simulink model "VCU_2023"  (Simulink 10.1)
settings: Solver=FixedStepDiscrete  StartTime=0.0  StopTime=10.0  FixedStep=0.001  RelTol=1e-3  EnableMultiTasking=on
PreLoadFcn:
  | try
  | MDL_setup;
  | catch
  | end
InitFcn:
  | EcoCoder_PreCheckLic();
undefined symbols (not defined in the file): APPS_max, APPS_min, BRK_TH, DiscIntNeverNeededParam
libraries: CoderSF_BSW_Libs x156, simulink x11
(part 1 of 2)
settings Model: Creator=HXL  LastModifiedBy=ecuri
settings Model: SuppressorTable=|
  | <?xml version="1.0" encoding="UTF-8" standalone="yes" ?>
  | <!DOCTYPE boost_serialization>
  | <boost_serialization signature="serialization::archive" version="17">
  | <DiagnosticSuppressor class_id="0" tracking_level="0" version="6">
  | 	<Table class_id="1" tracking_level="0" version="0">
  | 		<count>4</count>
  | 		<bucket_count>8</bucket_count>
  | 		<item_version>0</item_version>
  | 		<item class_id="2" tracking_level="0" version="0">
  | 			<first class_id="3" tracking_level="0" version="6">
  | 				<Source class_id="4" tracking_level="0" version="0">
  | 					<count>1</count>
  | 					<item_version>0</item_version>
  | 					<item>VCU_2023/Subsystem/CAN/Triggered Subsystem/N_R_Dec | M_R_Dec/Extract Bits1</item>
  | 				</Source>
  | 			</first>
  | 			<second class_id="5" tracking_level="0" version="6">
  | 				<SuppressedData class_id="6" tracking_level="0" version="0">
  | 					<count>2</count>
  | 					<bucket_count>8</bucket_count>
  | 					<item_version>0</item_version>
  | 					<item class_id="7" tracking_level="0" version="0">
  | 						<first class_id="8" tracking_level="0" version="6">
  | 							<ID>Simulink:DataType:WarningOverFlowDetected</ID>
  | 							<Cause>
  | 								<Source>
  | 									<count>0</count>
  | 									<item_version>0</item_version>
  | 								</Source>
  | 							</Cause>
  | 						</first>
  | 						<second class_id="9" tracking_level="0" version="6">
  | 							<Comment></Comment>
  | 							<User></User>
  | 							<LastModified class_id="10" tracking_level="0" version="0">
  | 								<ptime_date class_id="11" tracking_level="0" version="0">
  | 									<date>20160608</date>
  | 								</ptime_date>
  | 								<ptime_time_duration class_id="12" tracking_level="0" version="1">
  | 									<is_special>0</is_special>
  | 									<time_duration_hours>15</time_duration_hours>
  | 									<time_duration_minutes>43</time_duration_minutes>
  | 									<time_duration_seconds>6</time_duration_seconds>
  | 									<time_duration_fractional_seconds>0</time_duration_fractional_seconds>
  | 								</ptime_time_duration>
  | 							</LastModified>
  | 							<SuppressionType>1</SuppressionType>
  | 						</second>
  | 					</item>
  | 					<item>
  | 						<first>
  | 							<ID>SimulinkFixedPoint:util:Overflowoccurred</ID>
  | 							<Cause>
  | 								<Source>
  | 									<count>0</count>
  | 									<item_version>0</item_version>
  | 								</Source>
  | 							</Cause>
  | 						</first>
  | 						<second>
  | 							<Comment></Comment>
  | 							<User></User>
  | 							<LastModified>
  | 								<ptime_date>
  | 									<date>20160608</date>
  | 								</ptime_date>
  | 								<ptime_time_duration>
  | 									<is_special>0</is_special>
  | 									<time_duration_hours>15</time_duration_hours>
  | 									<time_duration_minutes>43</time_duration_minutes>
  | 									<time_duration_seconds>6</time_duration_seconds>
  | 									<time_duration_fractional_seconds>0</time_duration_fractional_seconds>
  | 								</ptime_time_duration>
  | 							</LastModified>
  | 							<SuppressionType>1</SuppressionType>
  | 						</second>
  | 					</item>
  | 				</SuppressedData>
  | 			</second>
  | 		</item>
  | 		<item>
  | 			<first>
  | 				<Source>
  | 					<count>1</count>
  | 					<item_version>0</item_version>
  | 					<item>VCU_2023/Subsystem/CAN/Triggered Subsystem/N_R_Dec | M_R_Dec/Extract Bits</item>
  | 				</Source>
  | 			</first>
  | 			<second>
  | 				<SuppressedData>
  | 					<count>2</count>
  | 					<bucket_count>8</bucket_count>
  | 					<item_version>0</item_version>
  | 					<item>
  | 						<first>
  | 							<ID>Simulink:DataType:WarningOverFlowDetected</ID>
  | 							<Cause>
  | 								<Source>
  | 									<count>0</count>
  | 									<item_version>0</item_version>
  | 								</Source>
  | 							</Cause>
  | 						</first>
  | 						<second>
  | 							<Comment></Comment>
  | 							<User></User>
  | 							<LastModified>
  | 								<ptime_date>
  | 									<date>20160608</date>
  | 								</ptime_date>
  | 								<ptime_time_duration>
  | 									<is_special>0</is_special>
  | 									<time_duration_hours>15</time_duration_hours>
  | 									<time_duration_minutes>43</time_duration_minutes>
  | 									<time_duration_seconds>6</time_duration_seconds>
  | 									<time_duration_fractional_seconds>0</time_duration_fractional_seconds>
  | 								</ptime_time_duration>
  | 							</LastModified>
  | 							<SuppressionType>1</SuppressionType>
  | 						</second>
  | 					</item>
  | 					<item>
  | 						<first>
  | 							<ID>SimulinkFixedPoint:util:Overflowoccurred</ID>
  | 							<Cause>
  | 								<Source>
  | 									<count>0</count>
  | 									<item_version>0</item_version>
  | 								</Source>
  | 							</Cause>
  | 						</first>
  | 						<second>
  | 							<Comment></Comment>
  | 							<User></User>
  | 							<LastModified>
  | 								<ptime_date>
  | 									<date>20160608</date>
  | 								</ptime_date>
  | 								<ptime_time_duration>
  | 									<is_special>0</is_special>
  | 									<time_duration_hours>15</time_duration_hours>
  | 									<time_duration_minutes>43</time_duration_minutes>
  | 									<time_duration_seconds>6</time_duration_seconds>
  | 									<time_duration_fractional_seconds>0</time_duration_fractional_seconds>
  | 								</ptime_time_duration>
  | 							</LastModified>
  | 							<SuppressionType>1</SuppressionType>
  | 						</second>
  | 					</item>
  | 				</SuppressedData>
  | 			</second>
  | 		</item>
  | 		<item>
  | 			<first>
  | 				<Source>
  | 					<count>1</count>
  | 					<item_version>0</item_version>
  | 					<item>VCU_2023/Subsystem/CAN/Triggered Subsystem/N_R_Acc | M R_Acc/Extract Bits1</item>
  | 				</Source>
  | 			</first>
  | 			<second>
  | 				<SuppressedData>
  | 					<count>2</count>
  | 					<bucket_count>8</bucket_count>
  | 					<item_version>0</item_version>
  | 					<item>
  | 						<first>
  | 							<ID>Simulink:DataType:WarningOverFlowDetected</ID>
  | 							<Cause>
  | 								<Source>
  | 									<count>0</count>
  | 									<item_version>0</item_version>
  | 								</Source>
  | 							</Cause>
  | 						</first>
  | 						<second>
  | 							<Comment></Comment>
  | 							<User></User>
  | 							<LastModified>
  | 								<ptime_date>
  | 									<date>20160608</date>
  | 								</ptime_date>
  | 								<ptime_time_duration>
  | 									<is_special>0</is_special>
  | 									<time_duration_hours>15</time_duration_hours>
  | 									<time_duration_minutes>43</time_duration_minutes>
  | 									<time_duration_seconds>6</time_duration_seconds>
  | 									<time_duration_fractional_seconds>0</time_duration_fractional_seconds>
  | 								</ptime_time_duration>
  | 							</LastModified>
  | 							<SuppressionType>1</SuppressionType>
  | 						</second>
  | 					</item>
  | 					<item>
  | 						<first>
  | 							<ID>SimulinkFixedPoint:util:Overflowoccurred</ID>
  | 							<Cause>
  | 								<Source>
  | 									<count>0</count>
  | 									<item_version>0</item_version>
  | 								</Source>
  | 							</Cause>
  | 						</first>
  | 						<second>
  | 							<Comment></Comment>
  | 							<User></User>
  | 							<LastModified>
  | 								<ptime_date>
  | 									<date>20160608</date>
  | 								</ptime_date>
  | 								<ptime_time_duration>
  | 									<is_special>0</is_special>
  | 									<time_duration_hours>15</time_duration_hours>
  | 									<time_duration_minutes>43</time_duration_minutes>
  | 									<time_duration_seconds>6</time_duration_seconds>
  | 									<time_duration_fractional_seconds>0</time_duration_fractional_seconds>
  | 								</ptime_time_duration>
  | 							</LastModified>
  | 							<SuppressionType>1</SuppressionType>
  | 						</second>
  | 					</item>
  | 				</SuppressedData>
  | 			</second>
  | 		</item>
  | 		<item>
  | 			<first>
  | 				<Source>
  | 					<count>1</count>
  | 					<item_version>0</item_version>
  | 					<item>VCU_2023/Subsystem/CAN/Triggered Subsystem/N_R_Acc | M R_Acc/Extract Bits</item>
  | 				</Source>
  | 			</first>
  | 			<second>
  | 				<SuppressedData>
  | 					<count>2</count>
  | 					<bucket_count>8</bucket_count>
  | 					<item_version>0</item_version>
  | 					<item>
  | 						<first>
  | 							<ID>Simulink:DataType:WarningOverFlowDetected</ID>
  | 							<Cause>
  | 								<Source>
  | 									<count>0</count>
  | 									<item_version>0</item_version>
  | 								</Source>
  | 							</Cause>
  | 						</first>
  | 						<second>
  | 							<Comment></Comment>
  | 							<User></User>
  | 							<LastModified>
  | 								<ptime_date>
  | 									<date>20160608</date>
  | 								</ptime_date>
  | 								<ptime_time_duration>
  | 									<is_special>0</is_special>
  | 									<time_duration_hours>15</time_duration_hours>
  | 									<time_duration_minutes>43</time_duration_minutes>
  | 									<time_duration_seconds>6</time_duration_seconds>
  | 									<time_duration_fractional_seconds>0</time_duration_fractional_seconds>
  | 								</ptime_time_duration>
  | 							</LastModified>
  | 							<SuppressionType>1</SuppressionType>
  | 						</second>
  | 					</item>
  | 					<item>
  | 						<first>
  | 							<ID>SimulinkFixedPoint:util:Overflowoccurred</ID>
  | 							<Cause>
  | 								<Source>
  | 									<count>0</count>
  | 									<item_version>0</item_version>
  | 								</Source>
  | 							</Cause>
  | 						</first>
  | 						<second>
  | 							<Comment></Comment>
  | 							<User></User>
  | 							<LastModified>
  | 								<ptime_date>
  | 									<date>20160608</date>
  | 								</ptime_date>
  | 								<ptime_time_duration>
  | 									<is_special>0</is_special>
  | 									<time_duration_hours>15</time_duration_hours>
  | 									<time_duration_minutes>43</time_duration_minutes>
  | 									<time_duration_seconds>6</time_duration_seconds>
  | 									<time_duration_fractional_seconds>0</time_duration_fractional_seconds>
  | 								</ptime_time_duration>
  | 							</LastModified>
  | 							<SuppressionType>1</SuppressionType>
  | 						</second>
  | 					</item>
  | 				</SuppressedData>
  | 			</second>
  | 		</item>
  | 	</Table>
  | </DiagnosticSuppressor>
  | 
  | </boost_serialization>
  | 
  | </boost_serialization>
settings DataIOCC: ExternalInput=InputData  SaveFormat=Structure  SignalLoggingSaveFormat=ModelDataLogs  SaveOutput=off  SignalLogging=off  DSMLogging=off  SaveTime=off
settings OptimizationCC: DefaultParameterBehavior=Inlined  InlineInvariantSignals=on  EnhancedBackFolding=on  StrengthReduction=on  EnableMemcpy=off  PassReuseOutputArgsAs=Individual arguments  ExpressionDepthLimit=2147483647  EfficientFloat2IntCast=on  LifeSpan=1  SimCompilerOptimization=on  OptimizeBlockOrder=speed  DifferentSizesBufferReuse=on  EfficientTunableParamExpr=on
settings DebuggingCC: AlgebraicLoopMsg=none  ArtificialAlgebraicLoopMsg=none  SaveWithDisabledLinksMsg=none  SaveWithParameterizedLinksMsg=none  CheckSSInitialOutputMsg=off  SignalResolutionControl=TryResolveAll  BlockPriorityViolationMsg=error  MinStepSizeMsg=none  InheritedTsInSrcMsg=none  MultiTaskDSMMsg=none  MultiTaskCondExecSysMsg=none  MultiTaskRateTransMsg=warning  TasksWithSamePriorityMsg=none  SigSpecEnsureSampleTimeMsg=none  IntegerOverflowMsg=error  Int32ToFloatConvMsg=none  ParameterPrecisionLossMsg=none  ParameterTunabilityLossMsg=none  FixptConstOverflowMsg=error  FcnCallInpInsideContextMsg=warning  UnconnectedInputMsg=error  UnconnectedOutputMsg=error  UnconnectedLineMsg=error  FrameProcessingCompatibilityMsg=none  BusObjectLabelMismatch=none  RootOutportRequireBusObject=none  UnknownTsInhSupMsg=none  ModelReferenceDataLoggingMessage=none  OperatingPointInterfaceChecksumMismatchMsg=none  SFUnusedDataAndEventsDiag=none  SFUnexpectedBacktrackingDiag=none  SFInvalidInputDataAccessInChartInitDiag=none  SFNoUnconditionalDefaultTransitionDiag=none  SFTransitionOutsideNaturalParentDiag=none  SFUnreachableExecutionPathDiag=none  IntegerSaturationMsg=error
settings HardwareCC: ProdLargestAtomicInteger=Long  ProdLargestAtomicFloat=Double  ProdIntDivRoundTo=Zero  ProdEndianess=BigEndian  ProdHWDeviceType=Freescale->MPC55xx  TargetIntDivRoundTo=Zero  TargetEndianess=BigEndian  TargetHWDeviceType=Freescale->MPC55xx
settings ModelReferenceCC: UpdateModelReferenceTargets=Force  ModelReferenceNumInstancesAllowed=Single
settings SFSimCC: SFSimEcho=off  SimBuildMode=sf_make_clean  MATLABDynamicMemAlloc=off
settings RTWCC: Description=Ecotrons MPC5xxx  SystemTargetFile=MPC5644A.tlc  GenerateMakefile=off  TemplateMakefile=ert_default_tmf  RTWVerbose=off  RetainRTWFile=on  RTWCompilerOptimization=on
settings CodeAppCC: IgnoreCustomStorageClasses=off  OperatorAnnotations=on  CustomSymbolStrGlobalVar=$N$M  CustomSymbolStrType=$N$M  CustomSymbolStrFcn=$N$M  CustomSymbolStrFcnArg=$N$M  CustomSymbolStrBlkIO=$N$M  CustomSymbolStrMacro=$N$M  StateflowObjectComments=off  InternalIdentifier=Classic
settings STFCustomTargetCC: CodeReplacementLibrary=ANSI_C  UtilityFuncGeneration=Shared location  MultiwordLength=256  IncludeMdlTerminateFcn=off  CombineOutputUpdateFcns=on  SuppressErrorStatus=on  ERTCustomFileBanners=on  SupportNonFinite=off  SupportComplex=off  SupportContinuousTime=off  SupportNonInlinedSFcns=off  MATLABClassNameForMDSCustomization=Simulink.SoftwareTarget.ERTCustomization  GRTInterface=off  SystemTargetFile=MPC5644A.tlc
settings ERTTargetCC: CodeReplacementLibrary=ANSI_C  UtilityFuncGeneration=Shared location  ParMdlRefBuildCompliant=off  CompOptLevelCompliant=off  ConcurrentExecutionCompliant=off  IncludeMdlTerminateFcn=off  SuppressErrorStatus=on  SupportNonFinite=off  SupportComplex=off  RemoveResetFunc=off  ModelStepFunctionPrototypeControlCompliant=off  CPPClassGenCompliant=off  UseToolchainInfoCompliant=off  GenerateASAP2=on  InlinedParameterPlacement=NonHierarchical  ERTCustomFileTemplate=MPC5644A_file_process.tlc  ERTFilePackagingFormat=Compact  PreserveIfCondition=on  ConvertIfToSwitch=off  PreserveExternInFcnDecls=off  SuppressUnreachableDefaultCases=off
settings CustomProperty: DataType=string  Value=EV2274A
settings EnumStrPairs: String=Removed
settings ConfigComp: DVMaxProcessTime=3600  DVDisplayUnsatisfiableObjectives=on  DVModelCoverageObjectives=MCDC  DVMaxTestCaseSteps=500  DVTestSuiteOptimization=CombinedObjectives  DVDetectActiveLogic=on

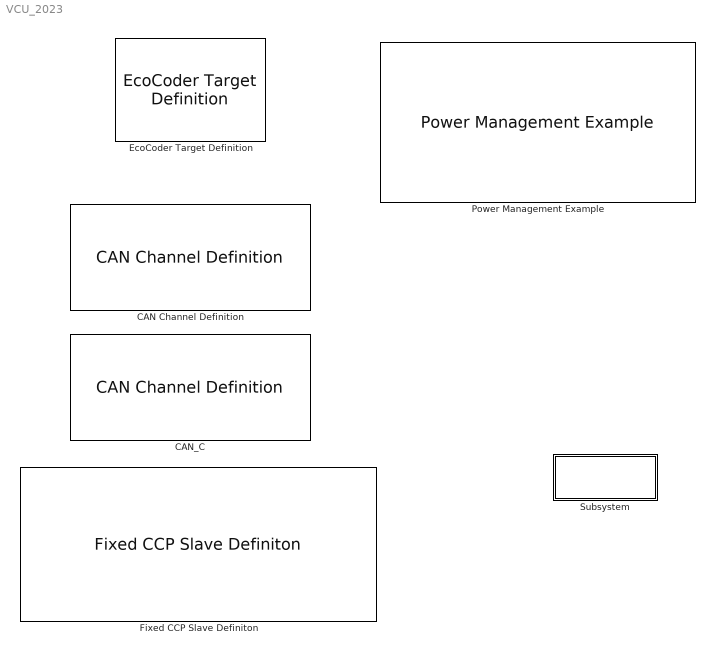
== system VCU_2023 ==
  CAN Channel Definition : CoderSF_BSW_Libs/CAN/CAN Channel Definition  channel=CAN_A  can_en=on  can_idfilter=off  can_rxextended=off  can_rxMask=hex2dec('7ff')  can_rxID=hex2dec('100')  can_baudrateIndex=500  can_txbuffer_size=30  can_rxbuffer_size=1  can_en_fd=off  nominalSamplePoint=7500  can_baudrateIndex_data=500  fastSamplePoint=7500  canfd_txbuffer_size=5  EcoCoderBlockID=C001_CANDef
  CAN_C : CoderSF_BSW_Libs/CAN/CAN Channel Definition  channel=CAN_C  can_en=on  can_idfilter=off  can_rxextended=off  can_rxMask=hex2dec('7ff')  can_rxID=hex2dec('100')  can_baudrateIndex=500  can_txbuffer_size=30  can_rxbuffer_size=1  can_en_fd=off  nominalSamplePoint=7500  can_baudrateIndex_data=500  fastSamplePoint=7500  canfd_txbuffer_size=5  EcoCoderBlockID=C001_CANDef
  EcoCoder Target Definition : CoderSF_BSW_Libs/EcoCoder Target Definition  targetECU=EV2274A  EcoCoderBlockID=T001_Target  enNoTriggerCall=on  flgBlockReduction=on  flgShowDebugDisp=off  flgDisTargetOutFIleCounter=off  flgClearAllOldFiles=on  tc275_cal_len=hex2dec('00008000')  internal_flash=[hex2dec('00020000'),hex2dec('000E0000')]  cal_rom_phy=[hex2dec('00010000'),hex2dec('00002000')]  cal_ram_wp=[hex2dec('4000F000'),hex2dec('00002000')]  cal_ram_msm=[hex2dec('40000000'),hex2dec('00002000')]  var_ram_wp=[hex2dec('40002000'),hex2dec('0000D000')]  write_back_fixed_ram=[hex2dec('40011000'),hex2dec('00001000')]  write_back_unfixed_ram=[hex2dec('40012000'),hex2dec('00001000')]  stack=[hex2dec('40013000'),hex2dec('00001000')]
      settings: AttributesFormatString=Target :%<targetECU>
  Fixed CCP Slave Definiton : CoderSF_BSW_Libs/CCP/Fixed CCP Slave Definiton  ccpType=Configurable  ccp_enSet=on  ccp_disASW=on  channel=CAN_A  stationaddressSet=hex2dec('0112')  croidSet=hex2dec('100')  dtoidSet=hex2dec('101')  daqidSet=[hex2dec('101') hex2dec('101') hex2dec('101') hex2dec('102')]  daqpidSet=[hex2dec('0') hex2dec('3C') hex2dec('78') hex2dec('0')]  daqlenSet=[hex2dec('0') hex2dec('20') hex2dec('30') hex2dec('30')]  daqperSet=[5 20 100 0]  EcoCoderBlockID=C002_CCPConf
  Power Management Example : CoderSF_BSW_Libs/System Management Blocks/Power Management Example  Priority=1  flgKeyFromIn=off  tKeyOffDelaySet=0.5  flgResetSWEnSet=1  tDbncKeyOffFallSet=0.1  tDbncKeyOffRiseSet=0.1  facAd2VoltSet=109/27846  uKeyOffThrSet=1  uKeyOnHystSet=1  flgCANRxLiveCheckEn=0  flgEnPwrDwnFailReset=0  flgNVMEn=on  tShtDwnWait=500  flgPwrDwnByEdgeTrigger=off  EcoCoderBlockID=PME001_Def
      settings: AttributesFormatString=Priority:%<Priority>
  Subsystem : Subsystem

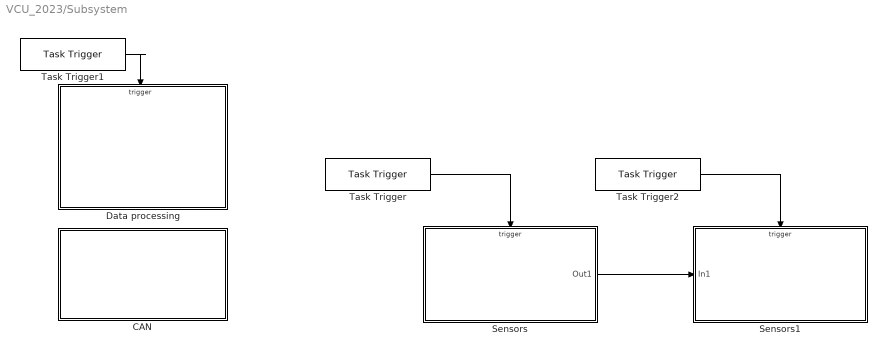
== system VCU_2023/Subsystem ==
  CAN : Subsystem
  Data processing : Subsystem
  Sensors : Subsystem
  Sensors1 : Subsystem
  Task Trigger : CoderSF_BSW_Libs/Task Scheduler/Task Trigger  tasktimeIndex=Task_H1ms
  Task Trigger1 : CoderSF_BSW_Libs/Task Scheduler/Task Trigger  Priority=1  tasktimeIndex=Task_L100ms  PrioritySet=1
  Task Trigger2 : CoderSF_BSW_Libs/Task Scheduler/Task Trigger  tasktimeIndex=Task_L50ms
  wires:
  Task Trigger/1 -> Sensors/Trigger
  Task Trigger1/1 -> Data processing/Trigger
  Task Trigger2/1 -> Sensors1/Trigger
  Sensors/1(Out1) -> Sensors1/1(In1)

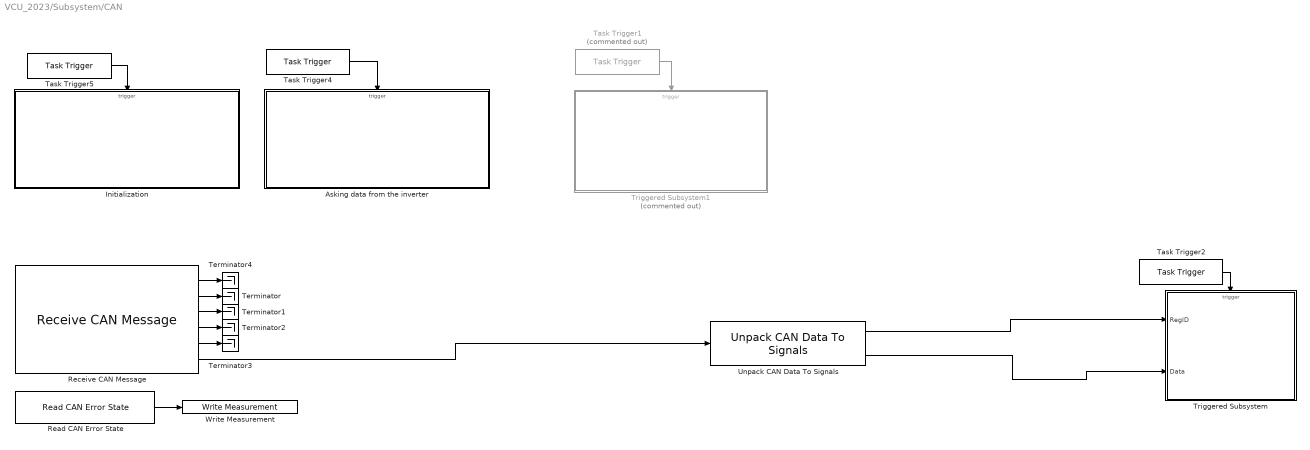
== system VCU_2023/Subsystem/CAN ==
  Asking data from the inverter : Subsystem
  Initialization : Subsystem
  Read CAN Error State : CoderSF_BSW_Libs/CAN/Read CAN Error State  channel=CAN_A
  Receive CAN Message : CoderSF_BSW_Libs/CAN/Receive CAN Message  channel=CAN_A  txid=hex2dec('181')  extended=off  txlen=5  tasktimeIndex=Task_L1ms
  Task Trigger1 : CoderSF_BSW_Libs/Task Scheduler/Task Trigger  Commented=on  tasktimeIndex=Task_L100ms
  Task Trigger2 : CoderSF_BSW_Libs/Task Scheduler/Task Trigger  Priority=2  tasktimeIndex=Task_L1ms  PrioritySet=2
  Task Trigger4 : CoderSF_BSW_Libs/Task Scheduler/Task Trigger  Priority=2  tasktimeIndex=Task_ini  PrioritySet=2
  Task Trigger5 : CoderSF_BSW_Libs/Task Scheduler/Task Trigger  Priority=1  tasktimeIndex=Task_ini  PrioritySet=1
  Terminator{,1..4} (5 alike) : Terminator
  Triggered Subsystem : Subsystem  TreatAsAtomicUnit=on
  Triggered Subsystem1 : Subsystem  Commented=on  TreatAsAtomicUnit=on
  Unpack CAN Data To Signals : CoderSF_BSW_Libs/CAN/Unpack CAN Data To Signals  Signal={{'RegID','DATA'},[0 8],[8 32],{'uint8','uint32'},{'Intel','Intel'}}
  Write Measurement : CoderSF_BSW_Libs/Calibration & Measurement/Write Measurement  variable_name=CAN_Error  variable_value=0  variable_type=uint8  numD=1  unitStr=""  descStr=""
      settings: AttributesFormatString=type:%<variable_type> Dimensions:%<numD>
  wires:
  Task Trigger4/1 -> Asking data from the inverter/Trigger
  Task Trigger1/1 -> Triggered Subsystem1/Trigger
  Unpack CAN Data To Signals/1 -> Triggered Subsystem/1(RegID)
  Unpack CAN Data To Signals/2 -> Triggered Subsystem/2(Data)
  Receive CAN Message/6 -> Unpack CAN Data To Signals/1
  Receive CAN Message/2 -> Terminator/1
  Receive CAN Message/3 -> Terminator1/1
  Receive CAN Message/4 -> Terminator2/1
  Receive CAN Message/5 -> Terminator3/1
  Task Trigger5/1 -> Initialization/Trigger
  Read CAN Error State/1 -> Write Measurement/1
  Task Trigger2/1 -> Triggered Subsystem/Trigger
  Receive CAN Message/1 -> Terminator4/1

== system VCU_2023/Subsystem/Data processing ==
  Trigger : TriggerPort  TriggerType=function-call  VariantControl=Variant  PortDimensions=1
  Electrical : Subsystem
  Temperature : Subsystem

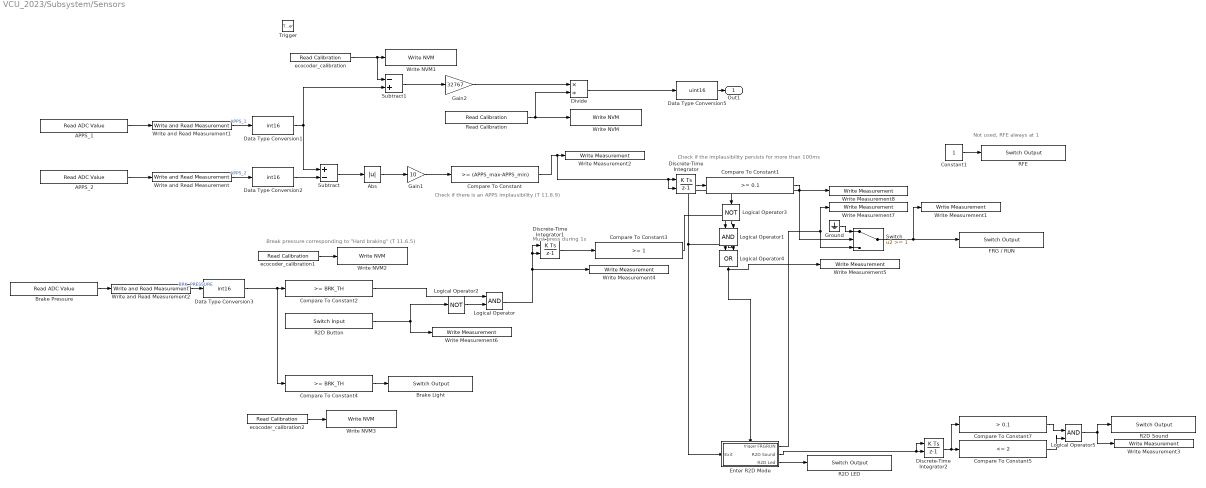
== system VCU_2023/Subsystem/Sensors ==
  note: Check if the implausibility persists for more than 100ms
  note: Check if there is an APPS implausibility (T 11.8.9)
  note: Not used, RFE always at 1
  note: Break pressure corresponding to "Hard braking" (T 11.6.5)
  note: Must press during 1s
  Trigger : TriggerPort  TriggerType=function-call  VariantControl=Variant  PortDimensions=1
  APPS_1 : CoderSF_BSW_Libs/ADC/Read ADC Value  channel=15
  APPS_2 : CoderSF_BSW_Libs/ADC/Read ADC Value  channel=19
  Abs : Abs
  Brake Light : CoderSF_BSW_Libs/Digital I//O/Switch Output  channel=LSO06
  Brake Pressure : CoderSF_BSW_Libs/ADC/Read ADC Value  channel=8
  Compare To Constant : simulink/Logic and Bit Operations/Compare To Constant  relop=>=  const=(APPS_max-APPS_min)  OutDataTypeStr=boolean
  Compare To Constant1 : simulink/Logic and Bit Operations/Compare To Constant  relop=>=  const=0.1  OutDataTypeStr=boolean
  Compare To Constant2 : simulink/Logic and Bit Operations/Compare To Constant  relop=>=  const=BRK_TH  OutDataTypeStr=boolean
  Compare To Constant3 : simulink/Logic and Bit Operations/Compare To Constant  relop=>=  const=1  OutDataTypeStr=boolean
  Compare To Constant4 : simulink/Logic and Bit Operations/Compare To Constant  relop=>=  const=BRK_TH  OutDataTypeStr=boolean
  Compare To Constant5 : simulink/Logic and Bit Operations/Compare To Constant  relop=<=  const=2  OutDataTypeStr=boolean
  Compare To Constant7 : simulink/Logic and Bit Operations/Compare To Constant  relop=>  const=0.1  OutDataTypeStr=boolean
  Constant1 : Constant  OutDataTypeStr=boolean
  Data Type Conversion1 : DataTypeConversion  OutDataTypeStr=int16
  Data Type Conversion2 : DataTypeConversion  OutDataTypeStr=int16
  Data Type Conversion3 : DataTypeConversion  OutDataTypeStr=int16
  Data Type Conversion5 : DataTypeConversion  OutDataTypeStr=uint16
  Discrete-Time Integrator : DiscreteIntegrator  ExternalReset=falling  SampleTime=-1  OutDataTypeStr=Inherit: Inherit via back propagation  UpperSaturationLimit=12  ICPrevOutput=DiscIntNeverNeededParam  ICPrevScaledInput=DiscIntNeverNeededParam
  Discrete-Time Integrator1 : DiscreteIntegrator  ExternalReset=falling  SampleTime=-1  OutDataTypeStr=Inherit: Inherit via back propagation  UpperSaturationLimit=12  ICPrevOutput=DiscIntNeverNeededParam  ICPrevScaledInput=DiscIntNeverNeededParam
  Discrete-Time Integrator2 : DiscreteIntegrator  ExternalReset=falling  SampleTime=-1  OutDataTypeStr=Inherit: Inherit via back propagation  UpperSaturationLimit=12  ICPrevOutput=DiscIntNeverNeededParam  ICPrevScaledInput=DiscIntNeverNeededParam
  Divide : Product  Inputs=*/
  Enter R2D Mode : Subsystem  TreatAsAtomicUnit=on
  FRG / RUN : CoderSF_BSW_Libs/Digital I//O/Switch Output  channel=HSO02
  Gain1 : Gain  Gain=10  OutDataTypeStr=int32
  Gain2 : Gain  Gain=32767  OutDataTypeStr=int32
  Ground : Ground
  Logical Operator : Logic  AllPortsSameDT=off  OutDataTypeStr=boolean
  Logical Operator1 : Logic  IconShape=distinctive  AllPortsSameDT=off  OutDataTypeStr=boolean
  Logical Operator2 : Logic  Operator=NOT  Inputs=1  IconShape=distinctive  AllPortsSameDT=off  OutDataTypeStr=boolean
  Logical Operator3 : Logic  Operator=NOT  Inputs=1  IconShape=distinctive  AllPortsSameDT=off  OutDataTypeStr=boolean
  Logical Operator4 : Logic  Operator=OR  IconShape=distinctive  AllPortsSameDT=off  OutDataTypeStr=boolean
  Logical Operator5 : Logic  IconShape=distinctive  AllPortsSameDT=off  OutDataTypeStr=boolean
  R2D Button : CoderSF_BSW_Libs/Digital I//O/Switch Input  portNum=DI01
  R2D LED : CoderSF_BSW_Libs/Digital I//O/Switch Output  channel=LSO08
  R2D Sound : CoderSF_BSW_Libs/Digital I//O/Switch Output  channel=LSO01
  RFE : CoderSF_BSW_Libs/Digital I//O/Switch Output  channel=HSO01
  Read Calibration : CoderSF_BSW_Libs/Calibration & Measurement/Read Calibration  variable_name=APPS_max  variable_value=4095  variable_type=int16  variable_min=[]  variable_max=[]  unitStr=""  descStr=""
      settings: AttributesFormatString=value:%<variable_value> type:%<variable_type> max:%<variable_max> Min:%<variable_min>
  Subtract : Sum  Inputs=+-
  Subtract1 : Sum  Inputs=-+
  Switch : Switch  Threshold=1  OutDataTypeStr=boolean
  Write Measurement1 : CoderSF_BSW_Libs/Calibration & Measurement/Write Measurement  variable_name=FRGRUN  variable_value=0  variable_type=boolean  numD=1  unitStr=""  descStr=""
      settings: AttributesFormatString=type:%<variable_type> Dimensions:%<numD>
  Write Measurement2 : CoderSF_BSW_Libs/Calibration & Measurement/Write Measurement  variable_name=APPS_implausibility  variable_value=0  variable_type=boolean  numD=1  unitStr=""  descStr=""
      settings: AttributesFormatString=type:%<variable_type> Dimensions:%<numD>
  Write Measurement3 : CoderSF_BSW_Libs/Calibration & Measurement/Write Measurement  variable_name=BUZZ  variable_value=0  variable_type=boolean  numD=1  unitStr=""  descStr=""
      settings: AttributesFormatString=type:%<variable_type> Dimensions:%<numD>
  Write Measurement4 : CoderSF_BSW_Libs/Calibration & Measurement/Write Measurement  variable_name=R2D  variable_value=0  variable_type=boolean  numD=1  unitStr=""  descStr=""
      settings: AttributesFormatString=type:%<variable_type> Dimensions:%<numD>
  Write Measurement5 : CoderSF_BSW_Libs/Calibration & Measurement/Write Measurement  variable_name=R2D2  variable_value=0  variable_type=boolean  numD=1  unitStr=""  descStr=""
      settings: AttributesFormatString=type:%<variable_type> Dimensions:%<numD>
  Write Measurement6 : CoderSF_BSW_Libs/Calibration & Measurement/Write Measurement  variable_name=R2D_btn  variable_value=0  variable_type=boolean  numD=1  unitStr=""  descStr=""
      settings: AttributesFormatString=type:%<variable_type> Dimensions:%<numD>
  Write Measurement7 : CoderSF_BSW_Libs/Calibration & Measurement/Write Measurement  variable_name=PREFRGRUN  variable_value=0  variable_type=boolean  numD=1  unitStr=""  descStr=""
      settings: AttributesFormatString=type:%<variable_type> Dimensions:%<numD>
  Write Measurement8 : CoderSF_BSW_Libs/Calibration & Measurement/Write Measurement  variable_name=APPS_PBM  variable_value=0  variable_type=boolean  numD=1  unitStr=""  descStr=""
      settings: AttributesFormatString=type:%<variable_type> Dimensions:%<numD>
  Write NVM : CoderSF_BSW_Libs/Non-volatile Memory Blocks/Write NVM  variable_name=nvmAPPS_max  flgDef=on  variable_value=0  variable_type=int16  variable_numD=1  unitStr=""  descStr=""  EcoCoderBlockID=N001_NVMVDEF
      settings: AttributesFormatString=value:%<variable_value> type:%<variable_type> D:%<variable_numD>
  Write NVM1 : CoderSF_BSW_Libs/Non-volatile Memory Blocks/Write NVM  variable_name=nvmAPPS_min  flgDef=on  variable_value=0  variable_type=int16  variable_numD=1  unitStr=""  descStr=""  EcoCoderBlockID=N001_NVMVDEF
      settings: AttributesFormatString=value:%<variable_value> type:%<variable_type> D:%<variable_numD>
  Write NVM2 : CoderSF_BSW_Libs/Non-volatile Memory Blocks/Write NVM  variable_name=nvmBRK_HARD_TH  flgDef=on  variable_value=0  variable_type=int16  variable_numD=1  unitStr=""  descStr=""  EcoCoderBlockID=N001_NVMVDEF
      settings: AttributesFormatString=value:%<variable_value> type:%<variable_type> D:%<variable_numD>
  Write NVM3 : CoderSF_BSW_Libs/Non-volatile Memory Blocks/Write NVM  variable_name=nvmBRK_TH  flgDef=on  variable_value=0  variable_type=int16  variable_numD=1  unitStr=""  descStr=""  EcoCoderBlockID=N001_NVMVDEF
      settings: AttributesFormatString=value:%<variable_value> type:%<variable_type> D:%<variable_numD>
  Write and Read Measurement : CoderSF_BSW_Libs/Calibration & Measurement/Write and Read Measurement  variable_name=APPS_2  variable_value=0  variable_type=uint16  numD=1  unitStr=""  descStr=""
      settings: AttributesFormatString=type:%<variable_type> Dimensions:%<numD>
  Write and Read Measurement1 : CoderSF_BSW_Libs/Calibration & Measurement/Write and Read Measurement  variable_name=APPS_1  variable_value=0  variable_type=uint16  numD=1  unitStr=""  descStr=""
      settings: AttributesFormatString=type:%<variable_type> Dimensions:%<numD>
  Write and Read Measurement2 : CoderSF_BSW_Libs/Calibration & Measurement/Write and Read Measurement  variable_name=BRK_PRESSURE  variable_value=0  variable_type=uint16  numD=1  unitStr=""  descStr=""
      settings: AttributesFormatString=type:%<variable_type> Dimensions:%<numD>
  ecocoder_calibration : CoderSF_BSW_Libs/Calibration & Measurement/Read Calibration  variable_name=APPS_min  variable_value=0  variable_type=int16  variable_min=[]  variable_max=[]  unitStr=""  descStr=""
      settings: AttributesFormatString=value:%<variable_value> type:%<variable_type> max:%<variable_max> Min:%<variable_min>
  ecocoder_calibration1 : CoderSF_BSW_Libs/Calibration & Measurement/Read Calibration  variable_name=BRK_HARD_TH  variable_value=0  variable_type=int16  variable_min=[]  variable_max=[]  unitStr=""  descStr=""
      settings: AttributesFormatString=value:%<variable_value> type:%<variable_type> max:%<variable_max> Min:%<variable_min>
  ecocoder_calibration2 : CoderSF_BSW_Libs/Calibration & Measurement/Read Calibration  variable_name=BRK_TH  variable_value=0  variable_type=int16  variable_min=[]  variable_max=[]  unitStr=""  descStr=""
      settings: AttributesFormatString=value:%<variable_value> type:%<variable_type> max:%<variable_max> Min:%<variable_min>
  Out1 : Outport
  wires:
  Compare To Constant/1 -> Discrete-Time Integrator/2, Discrete-Time Integrator/1, Write Measurement2/1
  Subtract/1 -> Abs/1
  APPS_2/1 -> Write and Read Measurement/1
  Abs/1 -> Gain1/1
  Gain1/1 -> Compare To Constant/1
  Divide/1 -> Data Type Conversion5/1
  Data Type Conversion1/1 -> Subtract1/2, Subtract/1
  Write and Read Measurement/1 -> Data Type Conversion2/1  "APPS_2"
  Data Type Conversion2/1 -> Subtract/2
  Read Calibration/1 -> Write NVM/1, Divide/2
  ecocoder_calibration/1 -> Subtract1/1, Write NVM1/1
  Subtract1/1 -> Gain2/1
  APPS_1/1 -> Write and Read Measurement1/1
  Write and Read Measurement1/1 -> Data Type Conversion1/1  "APPS_1"
  Gain2/1 -> Divide/1
  Compare To Constant1/1 -> Write Measurement8/1, Switch/2, Logical Operator4/1, Enter R2D Mode/1(Exit), Logical Operator3/1
  Discrete-Time Integrator/1 -> Compare To Constant1/1
  Switch/1 -> Write Measurement1/1, FRG / RUN/1
  Constant1/1 -> RFE/1
  Brake Pressure/1 -> Write and Read Measurement2/1
  Write and Read Measurement2/1 -> Data Type Conversion3/1  "BRK_PRESSURE"
  Data Type Conversion3/1 -> Compare To Constant4/1, Compare To Constant2/1
  ecocoder_calibration1/1 -> Write NVM2/1
  Compare To Constant2/1 -> Logical Operator/1
  Enter R2D Mode/1(FRGRUN) -> Switch/3, Write Measurement7/1
  Enter R2D Mode/3(R2D Led) -> R2D LED/1
  Discrete-Time Integrator1/1 -> Compare To Constant3/1
  Logical Operator/1 -> Write Measurement4/1, Discrete-Time Integrator1/1, Discrete-Time Integrator1/2
  Compare To Constant3/1 -> Logical Operator1/1
  ecocoder_calibration2/1 -> Write NVM3/1
  Compare To Constant4/1 -> Brake Light/1
  R2D Button/1 -> Write Measurement6/1, Logical Operator2/1
  Logical Operator2/1 -> Logical Operator/2
  Logical Operator3/1 -> Logical Operator1/2
  Logical Operator1/1 -> Logical Operator4/2
  Logical Operator4/1 -> Enter R2D Mode/Trigger, Write Measurement5/1
  Enter R2D Mode/2(R2D Sound) -> Discrete-Time Integrator2/1, Discrete-Time Integrator2/2
  Discrete-Time Integrator2/1 -> Compare To Constant7/1, Compare To Constant5/1
  Compare To Constant7/1 -> Logical Operator5/1
  Compare To Constant5/1 -> Logical Operator5/2
  Logical Operator5/1 -> Write Measurement3/1, R2D Sound/1
  Ground/1 -> Switch/1
  Data Type Conversion5/1 -> Out1/1

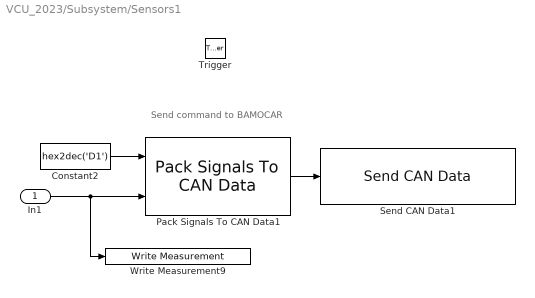
== system VCU_2023/Subsystem/Sensors1 ==
  note: Send command to BAMOCAR
  In1 : Inport
  Trigger : TriggerPort  TriggerType=function-call  VariantControl=Variant  PortDimensions=1
  Constant2 : Constant  Value=hex2dec('D1')  OutDataTypeStr=uint8
  Pack Signals To CAN Data1 : CoderSF_BSW_Libs/CAN/Pack Signals To CAN Data  Signal="{{'REG_90'  'Data1'},[0 8],[8 24],{'uint8'  'uint16'},{'Intel' 'Intel'}}"
  Send CAN Data1 : CoderSF_BSW_Libs/CAN/Send CAN Data  channel=CAN_A  txlen=3  txid="hex2dec(\"201\")"  frametype=Standard(11-bit ID)  showerror=off
  Write Measurement9 : CoderSF_BSW_Libs/Calibration & Measurement/Write Measurement  variable_name=TRQ_CMD_BAMOCAR  variable_value=0  variable_type=uint16  numD=1  unitStr=""  descStr=""
      settings: AttributesFormatString=type:%<variable_type> Dimensions:%<numD>
  wires:
  Pack Signals To CAN Data1/1 -> Send CAN Data1/1
  Constant2/1 -> Pack Signals To CAN Data1/1
  In1/1 -> Write Measurement9/1, Pack Signals To CAN Data1/2

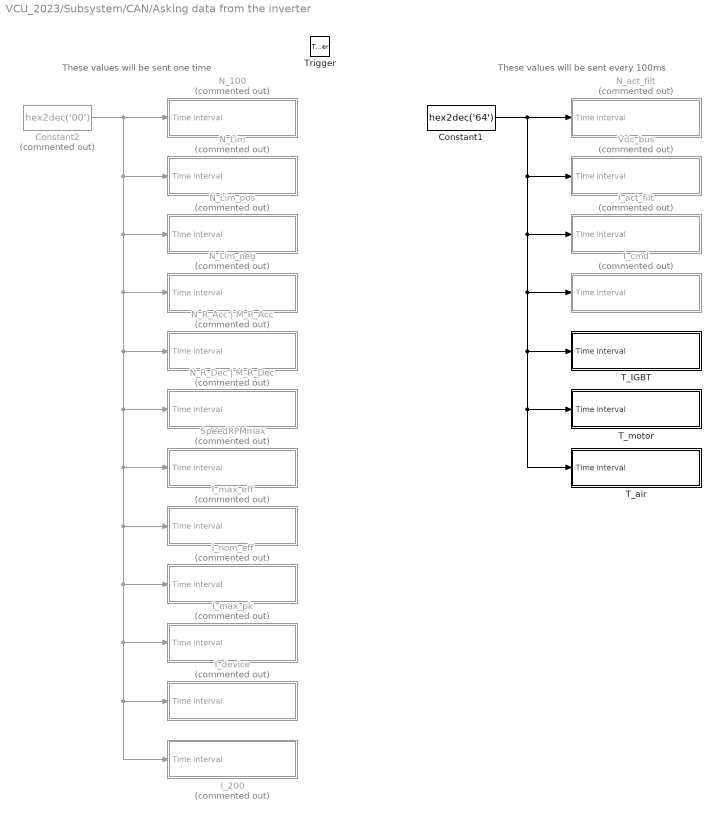
== system VCU_2023/Subsystem/CAN/Asking data from the inverter ==
  note: These values will be sent every 100ms
  note: These values will be sent one time
  Trigger : TriggerPort  TriggerType=function-call  VariantControl=Variant  PortDimensions=1
  Constant1 : Constant  Value=hex2dec('64')  OutDataTypeStr=uint8
  Constant2 : Constant  Commented=on  Value=hex2dec('00')  OutDataTypeStr=uint8
  I_200 : Subsystem  Commented=on
  I_act_filt : Subsystem  Commented=on
  I_cmd : Subsystem  Commented=on
  I_device : Subsystem  Commented=on
  I_max_eff : Subsystem  Commented=on
  I_max_pk : Subsystem  Commented=on
  I_nom_eff : Subsystem  Commented=on
  N_100 : Subsystem  Commented=on
  N_Lim : Subsystem  Commented=on
  N_Lim_neg : Subsystem  Commented=on
  N_Lim_pos : Subsystem  Commented=on
  N_R_Acc | M_R_Acc : Subsystem  Commented=on
  N_R_Dec | M_R_Dec : Subsystem  Commented=on
  N_act_filt : Subsystem  Commented=on
  SpeedRPMmax : Subsystem  Commented=on
  T_IGBT : Subsystem
  T_air : Subsystem
  T_motor : Subsystem
  Vdc_bus : Subsystem  Commented=on
  wires:
  Constant2/1 -> SpeedRPMmax/1(Time interval), I_200/1(Time interval), I_device/1(Time interval), I_max_pk/1(Time interval), I_nom_eff/1(Time interval), I_max_eff/1(Time interval), N_R_Dec | M_R_Dec/1(Time interval), N_R_Acc | M_R_Acc/1(Time interval), N_Lim_neg/1(Time interval), N_Lim_pos/1(Time interval), N_Lim/1(Time interval), N_100/1(Time interval)
  Constant1/1 -> T_air/1(Time interval), T_motor/1(Time interval), T_IGBT/1(Time interval), I_cmd/1(Time interval), I_act_filt/1(Time interval), Vdc_bus/1(Time interval), N_act_filt/1(Time interval)

== system VCU_2023/Subsystem/CAN/Initialization ==
  Trigger : TriggerPort  TriggerType=function-call  VariantControl=Variant  PortDimensions=1
  Constant : Constant  Value=0  OutDataTypeStr=boolean
  Constant1 : Constant  Value=0  OutDataTypeStr=boolean
  Disabling the inverter : Subsystem
  FRG/RUN : CoderSF_BSW_Libs/Digital I//O/Switch Output  channel=LSO07
  RFE : CoderSF_BSW_Libs/Digital I//O/Switch Output  channel=LSO06
  wires:
  Constant/1 -> RFE/1
  Constant1/1 -> FRG/RUN/1

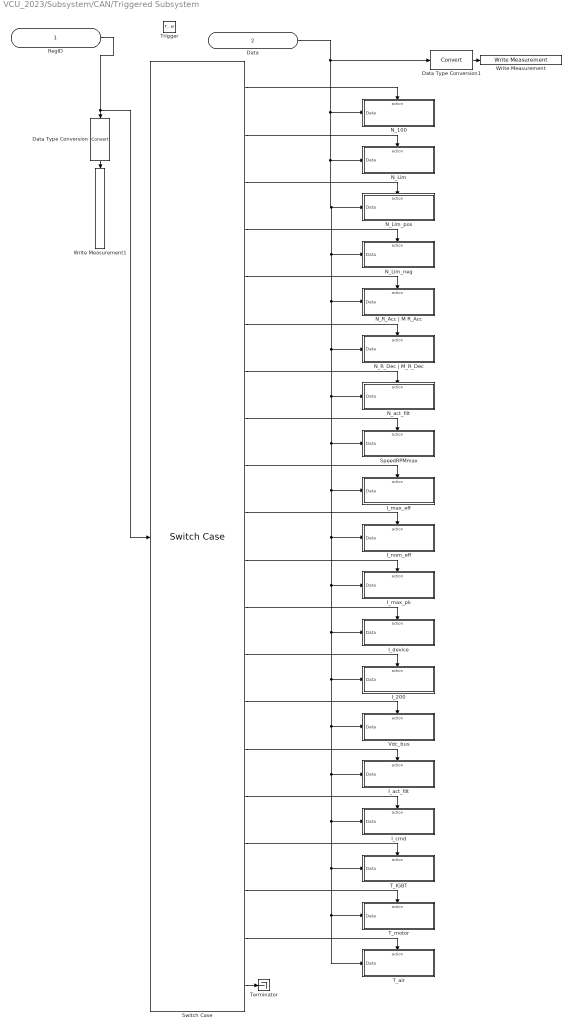
== system VCU_2023/Subsystem/CAN/Triggered Subsystem ==
  RegID : Inport
  Data : Inport  Port=2
  Trigger : TriggerPort  TriggerType=function-call  VariantControl=Variant
  Data Type Conversion : DataTypeConversion
  Data Type Conversion1 : DataTypeConversion
  I_200 : Subsystem  TreatAsAtomicUnit=on
  I_act_filt : Subsystem  TreatAsAtomicUnit=on
  I_cmd : Subsystem  TreatAsAtomicUnit=on
  I_device : Subsystem  TreatAsAtomicUnit=on
  I_max_eff : Subsystem  TreatAsAtomicUnit=on
  I_max_pk : Subsystem  TreatAsAtomicUnit=on
  I_nom_eff : Subsystem  TreatAsAtomicUnit=on
  N_100 : Subsystem  TreatAsAtomicUnit=on
  N_Lim : Subsystem  TreatAsAtomicUnit=on
  N_Lim_neg : Subsystem  TreatAsAtomicUnit=on
  N_Lim_pos : Subsystem  TreatAsAtomicUnit=on
  N_R_Acc | M R_Acc : Subsystem  TreatAsAtomicUnit=on
  N_R_Dec | M_R_Dec : Subsystem  TreatAsAtomicUnit=on
  N_act_filt : Subsystem  TreatAsAtomicUnit=on
  SpeedRPMmax : Subsystem  TreatAsAtomicUnit=on
  Switch Case : SwitchCase  CaseConditions={0xc8,0x34,0x3f,0x3e,0x35,0xed,0xce,0xa8,0x4d,0x4e,0xc4,0xc6,0xd9,0xeb,0x5f,0x26,0x4a,0x49,0x4b}
  T_IGBT : Subsystem  TreatAsAtomicUnit=on
  T_air : Subsystem  TreatAsAtomicUnit=on
  T_motor : Subsystem  TreatAsAtomicUnit=on
  Terminator : Terminator
  Vdc_bus : Subsystem  TreatAsAtomicUnit=on
  Write Measurement : CoderSF_BSW_Libs/Calibration & Measurement/Write Measurement  variable_name=DATA  variable_value=0  variable_type=int16  numD=1  unitStr=""  descStr=""
      settings: AttributesFormatString=type:%<variable_type> Dimensions:%<numD>
  Write Measurement1 : CoderSF_BSW_Libs/Calibration & Measurement/Write Measurement  variable_name=REGID  variable_value=0  variable_type=int16  numD=1  unitStr=""  descStr=""
      settings: AttributesFormatString=type:%<variable_type> Dimensions:%<numD>
  wires:
  Switch Case/15 -> I_act_filt/Action
  Data/1 -> Data Type Conversion1/1, T_air/1(Data), T_motor/1(Data), T_IGBT/1(Data), I_cmd/1(Data), I_act_filt/1(Data), Vdc_bus/1(Data), I_200/1(Data), I_device/1(Data), I_max_pk/1(Data), I_nom_eff/1(Data), I_max_eff/1(Data), SpeedRPMmax/1(Data), N_act_filt/1(Data), N_R_Dec | M_R_Dec/1(Data), N_R_Acc | M R_Acc/1(Data), N_Lim_neg/1(Data), N_Lim_pos/1(Data), N_Lim/1(Data), N_100/1(Data)
  Switch Case/17 -> T_IGBT/Action
  Switch Case/10 -> I_nom_eff/Action
  Switch Case/18 -> T_motor/Action
  Switch Case/5 -> N_R_Acc | M R_Acc/Action
  Switch Case/13 -> I_200/Action
  Switch Case/7 -> N_act_filt/Action
  Switch Case/16 -> I_cmd/Action
  Switch Case/11 -> I_max_pk/Action
  Switch Case/9 -> I_max_eff/Action
  Switch Case/6 -> N_R_Dec | M_R_Dec/Action
  Switch Case/8 -> SpeedRPMmax/Action
  Switch Case/14 -> Vdc_bus/Action
  Switch Case/1 -> N_100/Action
  Switch Case/4 -> N_Lim_neg/Action
  Switch Case/19 -> T_air/Action
  Switch Case/2 -> N_Lim/Action
  Switch Case/20 -> Terminator/1
  Switch Case/12 -> I_device/Action
  Switch Case/3 -> N_Lim_pos/Action
  Data Type Conversion/1 -> Write Measurement1/1
  RegID/1 -> Switch Case/1, Data Type Conversion/1
  Data Type Conversion1/1 -> Write Measurement/1

== system VCU_2023/Subsystem/CAN/Triggered Subsystem1 ==
  Trigger : TriggerPort  TriggerType=function-call  VariantControl=Variant  PortDimensions=1
  Constant : Constant  Value=0  OutDataTypeStr=uint8
  Pack Signals To CAN Data : CoderSF_BSW_Libs/CAN/Pack Signals To CAN Data  Signal="{{'Reg_Id' 'LVL_LV'  'LVL_HV' 'T_HV'},[0 8 16 24],[8 8 8 8],{'uint8'  'uint8' 'uint8' 'uint8'},{'Intel' 'Intel' 'Intel' 'Intel'}}"
  Send CAN Data : CoderSF_BSW_Libs/CAN/Send CAN Data  channel=CAN_C  txlen=3  txid=hex2dec('38')  frametype=Standard(11-bit ID)  showerror=off
  wires:
  Pack Signals To CAN Data/1 -> Send CAN Data/1
  Constant/1 -> Pack Signals To CAN Data/3, Pack Signals To CAN Data/2, Pack Signals To CAN Data/1, Pack Signals To CAN Data/4

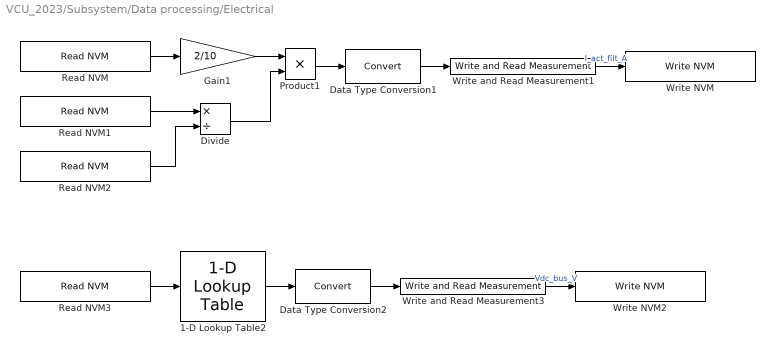
== system VCU_2023/Subsystem/Data processing/Electrical ==
  1-D Lookup Table2 : CoderSF_BSW_Libs/Calibration & Measurement/1-D Lookup Table  nam=Vdc_bus_V  breakpoint_type=int16  breakpoint_data=[0 748 1537 2327 3117 3906 4696 5485 6275 7065 7854 8644 9434 10223 11013 11802 12592 13382 14171 14961 15751 16540 17330 18119 18909 19699 20488 21278 22067 22857 23647 24436 25226 26016 26805 27595 28384 29174 29964 30753 31543 31751]  table_type=int16  table_data=[0 25 50 75 100 125 150 175 200 225 250 275 300 325 350 375 400 425 450 475 500 525 550 575 600 625 650 675 700 725 750 775 800 825 850 875 900 925 950 975 1000 1025]
  Data Type Conversion1 : DataTypeConversion
  Data Type Conversion2 : DataTypeConversion
  Divide : Product  Inputs=*/
  Gain1 : Gain  Gain=2/10
  Product1 : Product
  Read NVM : CoderSF_BSW_Libs/Non-volatile Memory Blocks/Read NVM  variable_name=nvmI_device  variable_type=Inherit from 'Variable definition'
  Read NVM1 : CoderSF_BSW_Libs/Non-volatile Memory Blocks/Read NVM  variable_name=nvmI_act_filt  variable_type=Inherit from 'Variable definition'
  Read NVM2 : CoderSF_BSW_Libs/Non-volatile Memory Blocks/Read NVM  variable_name=nvmI_200  variable_type=Inherit from 'Variable definition'
  Read NVM3 : CoderSF_BSW_Libs/Non-volatile Memory Blocks/Read NVM  variable_name=nvmVdc_bus  variable_type=Inherit from 'Variable definition'
  Write NVM : CoderSF_BSW_Libs/Non-volatile Memory Blocks/Write NVM  variable_name=nvmI_act_filt_A  flgDef=on  variable_value=0  variable_type=int16  variable_numD=1  unitStr=A  descStr=""  EcoCoderBlockID=N001_NVMVDEF
      settings: AttributesFormatString=value:%<variable_value> type:%<variable_type> D:%<variable_numD>
  Write NVM2 : CoderSF_BSW_Libs/Non-volatile Memory Blocks/Write NVM  variable_name=nvmVdc_bus_V  flgDef=on  variable_value=0  variable_type=int16  variable_numD=1  unitStr=V  descStr=""  EcoCoderBlockID=N001_NVMVDEF
      settings: AttributesFormatString=value:%<variable_value> type:%<variable_type> D:%<variable_numD>
  Write and Read Measurement1 : CoderSF_BSW_Libs/Calibration & Measurement/Write and Read Measurement  variable_name=I_act_filt_A  variable_value=0  variable_type=int16  numD=1  unitStr=A  descStr=""
      settings: AttributesFormatString=type:%<variable_type> Dimensions:%<numD>
  Write and Read Measurement3 : CoderSF_BSW_Libs/Calibration & Measurement/Write and Read Measurement  variable_name=Vdc_bus_V  variable_value=0  variable_type=int16  numD=1  unitStr=V  descStr=""
      settings: AttributesFormatString=type:%<variable_type> Dimensions:%<numD>
  wires:
  Product1/1 -> Data Type Conversion1/1
  Divide/1 -> Product1/2
  Read NVM2/1 -> Divide/2
  Gain1/1 -> Product1/1
  Read NVM1/1 -> Divide/1
  Data Type Conversion1/1 -> Write and Read Measurement1/1
  Read NVM/1 -> Gain1/1
  Write and Read Measurement1/1 -> Write NVM/1  "I_act_filt_A"
  1-D Lookup Table2/1 -> Data Type Conversion2/1
  Write and Read Measurement3/1 -> Write NVM2/1  "Vdc_bus_V"
  Data Type Conversion2/1 -> Write and Read Measurement3/1
  Read NVM3/1 -> 1-D Lookup Table2/1

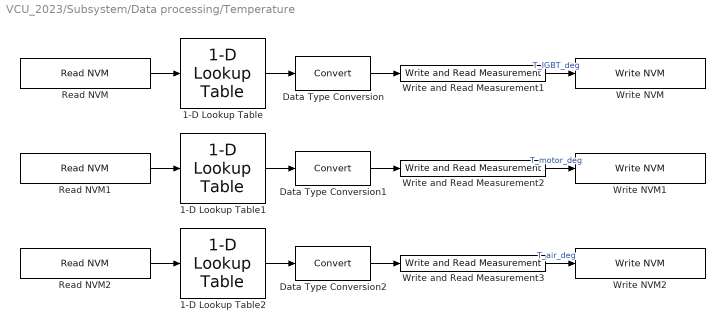
== system VCU_2023/Subsystem/Data processing/Temperature ==
  1-D Lookup Table : CoderSF_BSW_Libs/Calibration & Measurement/1-D Lookup Table  nam=T_IGBT_conversion  breakpoint_type=int16  breakpoint_data=[16245 16308 16387 16487 16609 16759 16938 17151 17400 17688 18017 18387 18797 19247 19733 20250 20793 21357 21933 22515 23097 23671 24232 24775 25296 25792 26261 26702 27114 27497 27851 28179 28480 28757 29011 29243 29456 29650 29827]  table_type=int16  table_data=[-35 -30 -25 -20 -15 -10 -5 0 5 10 15 20 25 30 35 40 45 50 55 60 65 70 75 80 85 90 95 100 105 110 115 120 125 130 135 140 145 150 155]
  1-D Lookup Table1 : CoderSF_BSW_Libs/Calibration & Measurement/1-D Lookup Table  nam=T_motor_conversion  breakpoint_type=int16  breakpoint_data=[7414 7687 7962 8240 8520 8802 9085 9369 9654 9939 10225 10510 10795 11080 11364 11646 11927 12207 12485 12762 13036 13308 13578 13846 14111 14373 14633 14890 15144 15391 15628 15852 16061 16251 16421 16569 16692 16789 16857]  table_type=int16  table_data=[-35 -30 -25 -20 -15 -10 -5 0 5 10 15 20 25 30 35 40 45 50 55 60 65 70 75 80 85 90 95 100 105 110 115 120 125 130 135 140 145 150 155]
  1-D Lookup Table2 : CoderSF_BSW_Libs/Calibration & Measurement/1-D Lookup Table  nam=T_air_conversion  breakpoint_type=int16  breakpoint_data=[8516 8785 9054 9322 9590 9857 10122 10386 10647 10907 11163 11418 11669 11917 12163 12404 12643 12878 13109 13337 13561 13781 13998 14210 14419 14624 14825 15022 15215]  table_type=int16  table_data=[-35 -30 -25 -20 -15 -10 -5 0 5 10 15 20 25 30 35 40 45 50 55 60 65 70 75 80 85 90 95 100 105]
  Data Type Conversion : DataTypeConversion
  Data Type Conversion1 : DataTypeConversion
  Data Type Conversion2 : DataTypeConversion
  Read NVM : CoderSF_BSW_Libs/Non-volatile Memory Blocks/Read NVM  variable_name=nvmT_IGBT  variable_type=Inherit from 'Variable definition'
  Read NVM1 : CoderSF_BSW_Libs/Non-volatile Memory Blocks/Read NVM  variable_name=nvmT_motor  variable_type=Inherit from 'Variable definition'
  Read NVM2 : CoderSF_BSW_Libs/Non-volatile Memory Blocks/Read NVM  variable_name=nvmT_air  variable_type=Inherit from 'Variable definition'
  Write NVM : CoderSF_BSW_Libs/Non-volatile Memory Blocks/Write NVM  variable_name=nvmT_IGBT_deg  flgDef=on  variable_value=0  variable_type=int16  variable_numD=1  unitStr=°C  descStr=""  EcoCoderBlockID=N001_NVMVDEF
      settings: AttributesFormatString=value:%<variable_value> type:%<variable_type> D:%<variable_numD>
  Write NVM1 : CoderSF_BSW_Libs/Non-volatile Memory Blocks/Write NVM  variable_name=nvmT_motor_deg  flgDef=on  variable_value=0  variable_type=int16  variable_numD=1  unitStr=°C  descStr=""  EcoCoderBlockID=N001_NVMVDEF
      settings: AttributesFormatString=value:%<variable_value> type:%<variable_type> D:%<variable_numD>
  Write NVM2 : CoderSF_BSW_Libs/Non-volatile Memory Blocks/Write NVM  variable_name=nvmT_air_deg  flgDef=on  variable_value=0  variable_type=int16  variable_numD=1  unitStr=°C  descStr=""  EcoCoderBlockID=N001_NVMVDEF
      settings: AttributesFormatString=value:%<variable_value> type:%<variable_type> D:%<variable_numD>
  Write and Read Measurement1 : CoderSF_BSW_Libs/Calibration & Measurement/Write and Read Measurement  variable_name=T_IGBT_deg  variable_value=0  variable_type=int16  numD=1  unitStr=°C  descStr=""
      settings: AttributesFormatString=type:%<variable_type> Dimensions:%<numD>
  Write and Read Measurement2 : CoderSF_BSW_Libs/Calibration & Measurement/Write and Read Measurement  variable_name=T_motor_deg  variable_value=0  variable_type=int16  numD=1  unitStr=°C  descStr=""
      settings: AttributesFormatString=type:%<variable_type> Dimensions:%<numD>
  Write and Read Measurement3 : CoderSF_BSW_Libs/Calibration & Measurement/Write and Read Measurement  variable_name=T_air_deg  variable_value=0  variable_type=int16  numD=1  unitStr=°C  descStr=""
      settings: AttributesFormatString=type:%<variable_type> Dimensions:%<numD>
  wires:
  Write and Read Measurement1/1 -> Write NVM/1  "T_IGBT_deg"
  Read NVM/1 -> 1-D Lookup Table/1
  Data Type Conversion/1 -> Write and Read Measurement1/1
  1-D Lookup Table/1 -> Data Type Conversion/1
  Data Type Conversion1/1 -> Write and Read Measurement2/1
  1-D Lookup Table1/1 -> Data Type Conversion1/1
  Read NVM1/1 -> 1-D Lookup Table1/1
  Write and Read Measurement2/1 -> Write NVM1/1  "T_motor_deg"
  Data Type Conversion2/1 -> Write and Read Measurement3/1
  1-D Lookup Table2/1 -> Data Type Conversion2/1
  Read NVM2/1 -> 1-D Lookup Table2/1
  Write and Read Measurement3/1 -> Write NVM2/1  "T_air_deg"

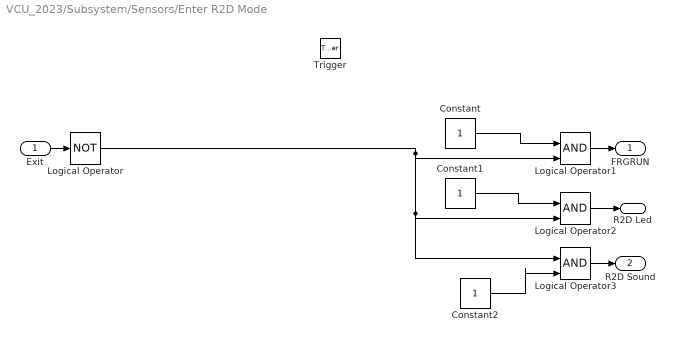
== system VCU_2023/Subsystem/Sensors/Enter R2D Mode ==
  Exit : Inport
  Trigger : TriggerPort  VariantControl=Variant  OutputDataType=int8  InitialTriggerSignalState=zero
  Constant : Constant  OutDataTypeStr=boolean
  Constant1 : Constant  OutDataTypeStr=boolean
  Constant2 : Constant  OutDataTypeStr=boolean
  Logical Operator : Logic  Operator=NOT  IconShape=distinctive  AllPortsSameDT=off  OutDataTypeStr=boolean
  Logical Operator1 : Logic  IconShape=distinctive  AllPortsSameDT=off  OutDataTypeStr=boolean
  Logical Operator2 : Logic  IconShape=distinctive  AllPortsSameDT=off  OutDataTypeStr=boolean
  Logical Operator3 : Logic  IconShape=distinctive  AllPortsSameDT=off  OutDataTypeStr=boolean
  FRGRUN : Outport
  R2D Sound : Outport  Port=2
  R2D Led : Outport  Port=3
  wires:
  Exit/1 -> Logical Operator/1
  Constant/1 -> Logical Operator1/1
  Logical Operator1/1 -> FRGRUN/1
  Logical Operator/1 -> Logical Operator3/1, Logical Operator2/2, Logical Operator1/2
  Logical Operator2/1 -> R2D Led/1
  Constant1/1 -> Logical Operator2/1
  Logical Operator3/1 -> R2D Sound/1
  Constant2/1 -> Logical Operator3/2

== system VCU_2023/Subsystem/CAN/Asking data from the inverter/I_200 ==
  Time interval : Inport
  Constant : Constant  Value=hex2dec('3d')  OutDataTypeStr=uint8
  Constant1 : Constant  Value=hex2dec('d9')  OutDataTypeStr=uint8
  Pack Signals To CAN Data : CoderSF_BSW_Libs/CAN/Pack Signals To CAN Data  Signal="{{'REG_31'  'Data1' 'Data2'},[0 8 16],[8 8 8],{'uint8'  'uint8' 'uint8'},{'Intel' 'Intel' 'Intel'}}"
  Send CAN Data : CoderSF_BSW_Libs/CAN/Send CAN Data  channel=CAN_A  txlen=3  txid=hex2dec('201')  frametype=Standard(11-bit ID)  showerror=off
  wires:
  Constant/1 -> Pack Signals To CAN Data/1
  Pack Signals To CAN Data/1 -> Send CAN Data/1
  Constant1/1 -> Pack Signals To CAN Data/2
  Time interval/1 -> Pack Signals To CAN Data/3

== system VCU_2023/Subsystem/CAN/Asking data from the inverter/I_act_filt ==
  Time interval : Inport
  Constant : Constant  Value=hex2dec('3d')  OutDataTypeStr=uint8
  Constant1 : Constant  Value=hex2dec('5f')  OutDataTypeStr=uint8
  Pack Signals To CAN Data : CoderSF_BSW_Libs/CAN/Pack Signals To CAN Data  Signal="{{'REG_31'  'Data1' 'Data2'},[0 8 16],[8 8 8],{'uint8'  'uint8' 'uint8'},{'Intel' 'Intel' 'Intel'}}"
  Send CAN Data : CoderSF_BSW_Libs/CAN/Send CAN Data  channel=CAN_A  txlen=3  txid=hex2dec('201')  frametype=Standard(11-bit ID)  showerror=off
  wires:
  Constant/1 -> Pack Signals To CAN Data/1
  Pack Signals To CAN Data/1 -> Send CAN Data/1
  Constant1/1 -> Pack Signals To CAN Data/2
  Time interval/1 -> Pack Signals To CAN Data/3

== system VCU_2023/Subsystem/CAN/Asking data from the inverter/I_cmd ==
  Time interval : Inport
  Constant : Constant  Value=hex2dec('3d')  OutDataTypeStr=uint8
  Constant1 : Constant  Value=hex2dec('26')  OutDataTypeStr=uint8
  Pack Signals To CAN Data : CoderSF_BSW_Libs/CAN/Pack Signals To CAN Data  Signal="{{'REG_31'  'Data1' 'Data2'},[0 8 16],[8 8 8],{'uint8'  'uint8' 'uint8'},{'Intel' 'Intel' 'Intel'}}"
  Send CAN Data : CoderSF_BSW_Libs/CAN/Send CAN Data  channel=CAN_A  txlen=3  txid=hex2dec('201')  frametype=Standard(11-bit ID)  showerror=off
  wires:
  Constant/1 -> Pack Signals To CAN Data/1
  Pack Signals To CAN Data/1 -> Send CAN Data/1
  Constant1/1 -> Pack Signals To CAN Data/2
  Time interval/1 -> Pack Signals To CAN Data/3
